simulink model "essaipid"  (R2016b)
settings: Solver=VariableStepAuto  StartTime=0.0  StopTime=10.0  FixedStep=0.001  MaxStep=0.001  RelTol=1e-3
settings Model: Creator=vanou  LastModifiedBy=vanou

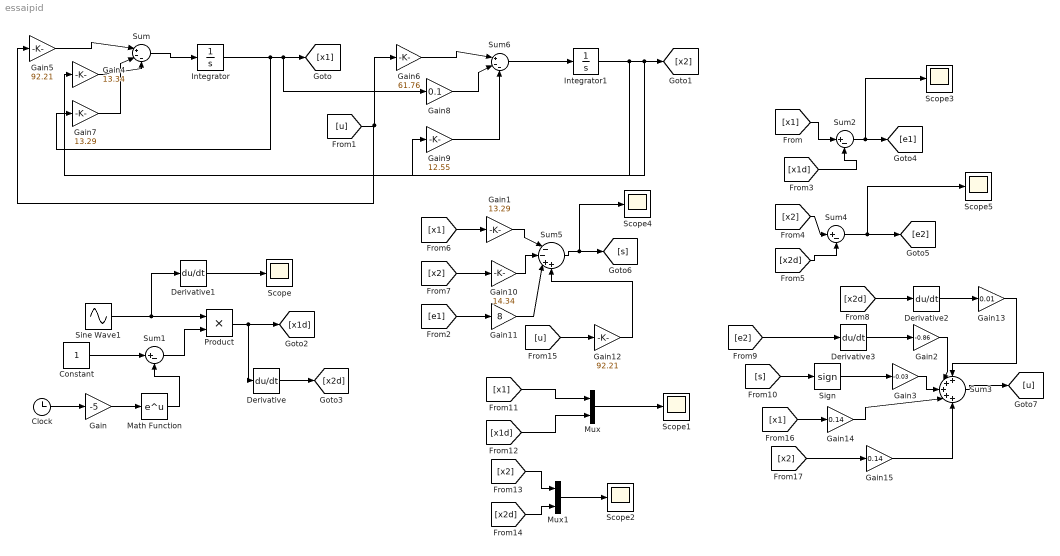
== system essaipid ==
  Clock : Clock
  Constant : Constant
  Derivative{,1..3} (4 alike) : Derivative
  Gain : Gain  Gain=-5
  Gain1 : Gain  Gain=13.29
  Gain10 : Gain  Gain=14.34
  Gain11 : Gain  Gain=8
  Gain12 : Gain  Gain=92.21
  Gain13 : Gain  Gain=0.01
  Gain14 : Gain  Gain=0.14
  Gain15 : Gain  Gain=0.14
  Gain2 : Gain  Gain=-0.86
  Gain3 : Gain  Gain=-0.03
  Gain4 : Gain  Gain=13.34
  Gain5 : Gain  Gain=92.21
  Gain6 : Gain  Gain=61.76
  Gain7 : Gain  Gain=13.29
  Gain8 : Gain  Gain=0.1
  Gain9 : Gain  Gain=12.55
  Integrator : Integrator
  Integrator1 : Integrator
  Math Function : Math  SaturateOnIntegerOverflow=on
  Mux : Mux  Inputs=2
  Mux1 : Mux  Inputs=2
  Product : Product
  Scope{,1..5} (6 alike) : Scope
  Sign : Signum
  Sine Wave1 : Sin  SampleTime=0
  Sum : Sum  Inputs=|+--
  Sum1 : Sum  Inputs=|+-
  Sum2 : Sum  Inputs=|+-
  Sum3 : Sum  Inputs=+++++
  Sum4 : Sum  Inputs=|+-
  Sum5 : Sum  Inputs=|--++
  Sum6 : Sum  Inputs=|+--
  wires:
  Clock/1 -> Gain/1
  Gain/1 -> Math Function/1
  Sine Wave1/1 -> Derivative1/1, Product/1
  Math Function/1 -> Sum1/2
  Constant/1 -> Sum1/1
  Sum1/1 -> Product/2
  Product/1 -> Derivative/1, [x1d]
  Derivative1/1 -> Scope/1
  [x1] -> Sum2/1
  [x1d] -> Sum2/2
  Sum2/1 -> Scope3/1, [e1]
  [x2] -> Sum4/1
  [x2d] -> Sum4/2
  Sum4/1 -> Scope5/1, [e2]
  Sum5/1 -> Scope4/1, [s]
  [x1] -> Gain1/1
  Gain1/1 -> Sum5/1
  [x2d] -> Derivative2/1
  Sum3/1 -> [u]
  Gain3/1 -> Sum3/3
  Gain2/1 -> Sum3/2
  Sign/1 -> Gain3/1
  [s] -> Sign/1
  [x1] -> Mux/1
  [x1d] -> Mux/2
  Mux/1 -> Scope1/1
  [x2] -> Mux1/1
  [x2d] -> Mux1/2
  Mux1/1 -> Scope2/1
  Derivative/1 -> [x2d]
  Sum/1 -> Integrator/1
  Gain5/1 -> Sum/1
  Gain7/1 -> Sum/2
  Gain4/1 -> Sum/3
  Sum6/1 -> Integrator1/1
  Gain6/1 -> Sum6/1
  Gain8/1 -> Sum6/2
  Integrator/1 -> Gain7/1, Gain8/1, [x1]
  Gain9/1 -> Sum6/3
  Integrator1/1 -> Gain9/1, Gain4/1, [x2]
  [u] -> Gain5/1, Gain6/1
  [x2] -> Gain10/1
  Gain10/1 -> Sum5/2
  [e1] -> Gain11/1
  Gain11/1 -> Sum5/3
  [u] -> Gain12/1
  Gain12/1 -> Sum5/4
  [e2] -> Derivative3/1
  Derivative3/1 -> Gain2/1
  Derivative2/1 -> Gain13/1
  Gain13/1 -> Sum3/1
  [x1] -> Gain14/1
  Gain14/1 -> Sum3/4
  [x2] -> Gain15/1
  Gain15/1 -> Sum3/5
